simulink model "f_cd_reorder"  (R2018a)
settings: Solver=VariableStepAuto  StartTime=0.0  StopTime=200000  RelTol=1e-3
libraries: xbsIndex_r4 x1711, casper_library_misc x12, xps_library x2, simulink x1
(part 4 of 9)

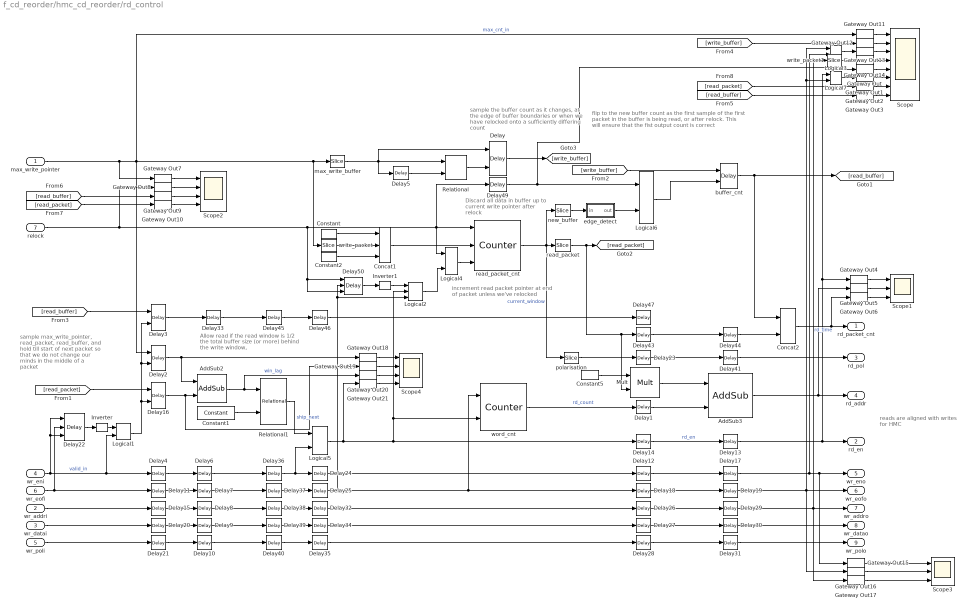
== system f_cd_reorder/hmc_cd_reorder/rd_control ==
  note: increment read packet pointer at
      | end of packet unless we've relocked
  note: flip to the new buffer count as the first sample of the
      | first packet in the buffer is being read, or after relock.
      | This will ensure that the fist output count is correct
  note: reads are aligned
      | with writes for HMC
  note: sample max_write_pointer,
      | read_packet, read_buffer,
      | and hold till start of
      | next packet so that
      | we do not change
      | our minds in the middle
      | of a packet
  note: sample the buffer count as it changes,
      | at the edge of buffer boundaries
      | or when we have relocked onto a
      | sufficiently differing count
  note: Allow read if the read window is 1/2
      | the total buffer size (or more)
      | behind the write window,
  note: Discard all data in buffer
      | up to current write pointer
      | after relock
  max_write_pointer : Inport
  wr_addri : Inport  Port=2
  wr_datai : Inport  Port=3
  wr_eni : Inport  Port=4
  wr_poli : Inport  Port=5
  wr_eofi : Inport  Port=6
  relock : Inport  Port=7
  AddSub2 : xbsIndex_r4/AddSub  mode=Subtraction  use_carryin=off  use_carryout=off  en=off  latency=1  precision=User Defined  arith_type=Unsigned  n_bits=n_bits_packets  bin_pt=0  quantization=Truncate  overflow=Wrap  use_behavioral_HDL=on  hw_selection=Fabric  pipelined=off  use_rpm=on  dbl_ovrd=off  block_type=addsub
      settings: xl_area=[0, 0, 0, 0, 0, 0, 0]  block_version=10.1.3
  AddSub3 : xbsIndex_r4/AddSub  mode=Addition  use_carryin=off  use_carryout=off  en=off  latency=1  precision=User Defined  arith_type=Unsigned  n_bits=n_bits_buffer_size-1  bin_pt=0  quantization=Truncate  overflow=Wrap  use_behavioral_HDL=on  hw_selection=Fabric  pipelined=off  use_rpm=on  dbl_ovrd=off  block_type=addsub
      settings: xl_area=[0, 0, 0, 0, 0, 0, 0]  block_version=10.1.3
  Concat1 : xbsIndex_r4/Concat  num_inputs=3  dbl_ovrd=off  block_type=concat
      settings: block_version=10.1.3
  Concat2 : xbsIndex_r4/Concat  num_inputs=2  dbl_ovrd=off  block_type=concat
      settings: block_version=10.1.3
  Constant : xbsIndex_r4/Constant  const=0  gui_display_data_type=Fixed-point  arith_type=Unsigned  n_bits=1  bin_pt=0  preci_type=Single  exp_width=8  frac_width=24  explicit_period=on  period=1  equ=P=C  opselect=C  inp2=PCIN>>17  opr=+  inp1=P  carry=CIN  dbl_ovrd=off  block_type=constant
  Constant1 : xbsIndex_r4/Constant  const=2^(n_bits_packets - 1)  gui_display_data_type=Fixed-point  arith_type=Unsigned  n_bits=n_bits_packets  bin_pt=0  preci_type=Single  exp_width=8  frac_width=24  explicit_period=on  period=1  equ=P=C  opselect=C  inp2=PCIN>>17  opr=+  inp1=P  carry=CIN  dbl_ovrd=off  block_type=constant
  Constant2 : xbsIndex_r4/Constant  const=0  gui_display_data_type=Fixed-point  arith_type=Unsigned  n_bits=1  bin_pt=0  preci_type=Single  exp_width=8  frac_width=24  explicit_period=on  period=1  equ=P=C  opselect=C  inp2=PCIN>>17  opr=+  inp1=P  carry=CIN  dbl_ovrd=off  block_type=constant
  Constant5 : xbsIndex_r4/Constant  const=packet_size  gui_display_data_type=Fixed-point  arith_type=Unsigned  n_bits=ceil(log2(packet_size))+1  bin_pt=0  preci_type=Single  exp_width=8  frac_width=24  explicit_period=on  period=1  equ=P=C  opselect=C  inp2=PCIN>>17  opr=+  inp1=P  carry=CIN  dbl_ovrd=off  block_type=constant
  Delay{,2..3,16} (4 alike) : xbsIndex_r4/Delay  rst=off  infoeditControl=Selection of Reset will increase slice count due to use of real FFs and instead of SRLs  en=on  latency=1  reg_retiming=on  dbl_ovrd=off  block_type=delay
      Delay16 settings: xl_area=[0, 0, 0, 0, 0, 0, 0]
      Delay2 settings: xl_area=[0, 0, 0, 0, 0, 0, 0]
      Delay3 settings: xl_area=[0, 0, 0, 0, 0, 0, 0]
  Delay{1,12,14,18,23,26..28,43,47} (10 alike) : xbsIndex_r4/Delay  rst=off  infoeditControl=Selection of Reset will increase slice count due to use of real FFs and instead of SRLs  en=off  latency=2  reg_retiming=on  dbl_ovrd=off  block_type=delay
      settings: xl_area=[0, 0, 0, 0, 0, 0, 0]
  Delay{4..11,13,15,17,19..21,24..25,29..41,44..46,49} (33 alike) : xbsIndex_r4/Delay  rst=off  infoeditControl=Selection of Reset will increase slice count due to use of real FFs and instead of SRLs  en=off  latency=1  reg_retiming=on  dbl_ovrd=off  block_type=delay
      Delay10 settings: xl_area=[0, 0, 0, 0, 0, 0, 0]
      Delay11 settings: xl_area=[0, 0, 0, 0, 0, 0, 0]
      Delay13 settings: infoedit=Hardware notes: A delay line is a chain, each link of which is an SRL16 or SRL32 followed by a flip-flop.  xl_area=[0, 0, 0, 0, 0, 0, 0]
      Delay15 settings: xl_area=[0, 0, 0, 0, 0, 0, 0]
      Delay17 settings: infoedit=Hardware notes: A delay line is a chain, each link of which is an SRL16 or SRL32 followed by a flip-flop.  xl_area=[0, 0, 0, 0, 0, 0, 0]
      Delay19 settings: infoedit=Hardware notes: A delay line is a chain, each link of which is an SRL16 or SRL32 followed by a flip-flop.  xl_area=[0, 0, 0, 0, 0, 0, 0]
      Delay20 settings: xl_area=[0, 0, 0, 0, 0, 0, 0]
      Delay21 settings: xl_area=[0, 0, 0, 0, 0, 0, 0]
      Delay24 settings: xl_area=[0, 0, 0, 0, 0, 0, 0]
      Delay25 settings: xl_area=[0, 0, 0, 0, 0, 0, 0]
      Delay29 settings: infoedit=Hardware notes: A delay line is a chain, each link of which is an SRL16 or SRL32 followed by a flip-flop.  xl_area=[0, 0, 0, 0, 0, 0, 0]
      Delay30 settings: infoedit=Hardware notes: A delay line is a chain, each link of which is an SRL16 or SRL32 followed by a flip-flop.  xl_area=[0, 0, 0, 0, 0, 0, 0]
      Delay31 settings: infoedit=Hardware notes: A delay line is a chain, each link of which is an SRL16 or SRL32 followed by a flip-flop.  xl_area=[0, 0, 0, 0, 0, 0, 0]
      Delay32 settings: xl_area=[0, 0, 0, 0, 0, 0, 0]
      Delay33 settings: xl_area=[0, 0, 0, 0, 0, 0, 0]
      Delay34 settings: xl_area=[0, 0, 0, 0, 0, 0, 0]
      Delay35 settings: xl_area=[0, 0, 0, 0, 0, 0, 0]
      Delay36 settings: xl_area=[0, 0, 0, 0, 0, 0, 0]
      Delay37 settings: xl_area=[0, 0, 0, 0, 0, 0, 0]
      Delay38 settings: xl_area=[0, 0, 0, 0, 0, 0, 0]
      Delay39 settings: xl_area=[0, 0, 0, 0, 0, 0, 0]
      Delay4 settings: xl_area=[0, 0, 0, 0, 0, 0, 0]
      Delay40 settings: xl_area=[0, 0, 0, 0, 0, 0, 0]
      Delay41 settings: infoedit=Hardware notes: A delay line is a chain, each link of which is an SRL16 or SRL32 followed by a flip-flop.  xl_area=[0, 0, 0, 0, 0, 0, 0]
      Delay44 settings: infoedit=Hardware notes: A delay line is a chain, each link of which is an SRL16 or SRL32 followed by a flip-flop.  xl_area=[0, 0, 0, 0, 0, 0, 0]
      Delay45 settings: xl_area=[0, 0, 0, 0, 0, 0, 0]
      Delay46 settings: xl_area=[0, 0, 0, 0, 0, 0, 0]
      Delay49 settings: xl_area=[0, 0, 0, 0, 0, 0, 0]
      Delay5 settings: xl_area=[0, 0, 0, 0, 0, 0, 0]
      Delay6 settings: xl_area=[0, 0, 0, 0, 0, 0, 0]
      Delay7 settings: xl_area=[0, 0, 0, 0, 0, 0, 0]
      Delay8 settings: xl_area=[0, 0, 0, 0, 0, 0, 0]
      Delay9 settings: xl_area=[0, 0, 0, 0, 0, 0, 0]
  Delay22 : xbsIndex_r4/Delay  rst=on  infoeditControl=Selection of Reset will increase slice count due to use of real FFs and instead of SRLs  en=on  latency=1  reg_retiming=on  dbl_ovrd=off  block_type=delay
      settings: xl_area=[0, 0, 0, 0, 0, 0, 0]
  Delay50 : xbsIndex_r4/Delay  rst=on  infoeditControl=Selection of Reset will increase slice count due to use of real FFs and instead of SRLs  en=on  latency=1  reg_retiming=on  dbl_ovrd=off  block_type=delay
      settings: xl_area=[0, 0, 0, 0, 0, 0, 0]
  Gateway Out{,1..21} (22 alike) : xbsIndex_r4/Gateway Out  inherit_from_input=off  hdl_port=off  rows=1  columns=1  UseAsDAC=off  DACChannel='1'  interface=None  automatic_assignment=on  address_offset=hex2dec('00')  intf_name=''  intf_description=''  timing_constraint=None  locs_specified=off  LOCs={}  io_standard={}  block_type=gatewayout
  Inverter : xbsIndex_r4/Inverter  en=off  latency=0  dbl_ovrd=off  block_type=inv
  Inverter1 : xbsIndex_r4/Inverter  en=off  latency=0  dbl_ovrd=off  block_type=inv
  Logical1 : xbsIndex_r4/Logical  logical_function=AND  inputs=2  en=off  latency=0  precision=Full  arith_type=Unsigned  n_bits=8  bin_pt=2  align_bp=on  dbl_ovrd=off  block_type=logical
      settings: xl_area=[0, 0, 0, 0, 0, 0, 0]
  Logical2 : xbsIndex_r4/Logical  logical_function=AND  inputs=3  en=off  latency=0  precision=Full  arith_type=Unsigned  n_bits=8  bin_pt=2  align_bp=on  dbl_ovrd=off  block_type=logical
      settings: xl_area=[0, 0, 0, 0, 0, 0, 0]
  Logical3 : xbsIndex_r4/Logical  logical_function=AND  inputs=2  en=off  latency=0  precision=Full  arith_type=Unsigned  n_bits=8  bin_pt=2  align_bp=on  dbl_ovrd=off  block_type=logical
      settings: xl_area=[0, 0, 0, 0, 0, 0, 0]
  Logical4 : xbsIndex_r4/Logical  logical_function=OR  inputs=2  en=off  latency=0  precision=Full  arith_type=Unsigned  n_bits=8  bin_pt=2  align_bp=on  dbl_ovrd=off  block_type=logical
      settings: xl_area=[0, 0, 0, 0, 0, 0, 0]
  Logical5 : xbsIndex_r4/Logical  logical_function=AND  inputs=2  en=off  latency=1  precision=Full  arith_type=Unsigned  n_bits=8  bin_pt=2  align_bp=on  dbl_ovrd=off  block_type=logical
      settings: xl_area=[0, 0, 0, 0, 0, 0, 0]
  Logical6 : xbsIndex_r4/Logical  logical_function=OR  inputs=2  en=off  latency=2  precision=Full  arith_type=Unsigned  n_bits=8  bin_pt=2  align_bp=on  dbl_ovrd=off  block_type=logical
      settings: xl_area=[0, 0, 0, 0, 0, 0, 0]
  Logical7 : xbsIndex_r4/Logical  logical_function=AND  inputs=2  en=off  latency=0  precision=Full  arith_type=Unsigned  n_bits=8  bin_pt=2  align_bp=on  dbl_ovrd=off  block_type=logical
      settings: xl_area=[0, 0, 0, 0, 0, 0, 0]
  Mult : xbsIndex_r4/Mult  precision=User Defined  arith_type=Unsigned  n_bits=n_bits_buffer_size-1  bin_pt=0  quantization=Truncate  overflow=Wrap  en=off  latency=2  use_behavioral_HDL=on  opt=Speed  use_embedded=on  optimum_pipeline=off  pipeline=on  dbl_ovrd=off  use_rpm=on  placement_style=Triangular  block_type=mult
  Relational : xbsIndex_r4/Relational  mode=a!=b  op_type=Bool  en=off  latency=0  dbl_ovrd=off  block_type=relational
  Relational1 : xbsIndex_r4/Relational  mode=a>=b  op_type=Bool  en=off  latency=1  dbl_ovrd=off  block_type=relational
      settings: xl_area=[0, 0, 0, 0, 0, 0, 0]  block_version=10.1.3
  Scope : Scope  NumInputPorts=8
  Scope1 : Scope  NumInputPorts=3
  Scope2 : Scope  NumInputPorts=4
  Scope3 : Scope  NumInputPorts=3
  Scope4 : Scope  NumInputPorts=4
  buffer_cnt : xbsIndex_r4/Delay  rst=off  infoeditControl=Selection of Reset will increase slice count due to use of real FFs and instead of SRLs  en=on  latency=1  reg_retiming=on  dbl_ovrd=off  block_type=delay
  edge_detect : Subsystem  AncestorBlock=casper_library_misc/edge_detect  mask(edge_detect){edge=Both, polarity=Active High, x_in=[0 0.08 0.08 0.16 0.16 0.24 0.24 0.32 0.32 0.4], y_in=[-1 -1  1  1  1  1  1  1  1  1], x_out=[0.6 0.68 0.68 0.76 0.76 0.84 0.84 0.92 0.92 1], y_out=[-1 -1  1  1 -1 -1 -1 -1 -1 -1]}
      mask prompts: edge "Edge Type"; polarity "Output Polarity"; x_in "Input X Positions"; y_in "Input Y Positions"; x_out "Output X Positions"; y_out "Output Y Positions"
      mask help: Output is active for one-cycle after each edge of the specified type (i.e. rising, falling or both).
      mask init: same as f_cd_reorder/data_width_convert/edge_detect
      settings: AttributesFormatString=|
      | both edges
      | active high
      mask Help: Output is active for one-cycle after each edge of the specified type (i.e. rising, falling, or both).  Latency is zero.
      mask TypeOptions edge: Rising | Falling | Both
      mask TypeOptions polarity: Active High | Active Low
      mask Display:
      | plot(x_in_num,0.5+y_in_num*0.2);
      | plot(x_out_num,0.5+y_out_num*0.2);
  max_write_buffer : xbsIndex_r4/Slice  nbits=1  boolean_output=off  mode=Two Bit Locations  bit1=0  base1=MSB of Input  bit0=n_bits_packets  base0=LSB of Input  dbl_ovrd=off  block_type=slice
      settings: block_version=10.1.3
  new_buffer : xbsIndex_r4/Slice  nbits=1  boolean_output=on  mode=Upper Bit Location + Width  bit1=0  base1=MSB of Input  bit0=0  base0=LSB of Input  dbl_ovrd=off  block_type=slice
  polarisation : xbsIndex_r4/Slice  nbits=1  boolean_output=off  mode=Lower Bit Location + Width  bit1=0  base1=MSB of Input  bit0=0  base0=LSB of Input  dbl_ovrd=off  block_type=slice
  read_packet : xbsIndex_r4/Slice  nbits=n_bits_packets  boolean_output=off  mode=Lower Bit Location + Width  bit1=0  base1=MSB of Input  bit0=1  base0=LSB of Input  dbl_ovrd=off  block_type=slice
  read_packet_cnt : xbsIndex_r4/Counter  cnt_type=Free Running  cnt_to=Inf  operation=Up  start_count=0  cnt_by_val=1  arith_type=Unsigned  n_bits=1+n_bits_packets+1  bin_pt=0  load_pin=on  rst=off  en=on  explicit_period=off  period=1  use_behavioral_HDL=off  implementation=Fabric  use_rpm=on  dbl_ovrd=off  block_type=counter
      settings: xl_area=[0, 0, 0, 0, 0, 0, 0]
  word_cnt : xbsIndex_r4/Counter  cnt_type=Count Limited  cnt_to=packet_size-1  operation=Up  start_count=0  cnt_by_val=1  arith_type=Unsigned  n_bits=ceil(log2(packet_size))  bin_pt=0  load_pin=off  rst=on  en=on  explicit_period=off  period=1  use_behavioral_HDL=on  implementation=Fabric  use_rpm=on  dbl_ovrd=off  block_type=counter
      settings: xl_area=[0, 0, 0, 0, 0, 0, 0]
  write_packet : xbsIndex_r4/Slice  nbits=n_bits_packets  boolean_output=off  mode=Lower Bit Location + Width  bit1=0  base1=MSB of Input  bit0=0  base0=LSB of Input  dbl_ovrd=off  block_type=slice
      settings: block_version=10.1.3
  write_packet1 : xbsIndex_r4/Slice  nbits=n_bits_packets  boolean_output=off  mode=Lower Bit Location + Width  bit1=0  base1=MSB of Input  bit0=ceil(log2(packet_size))  base0=LSB of Input  dbl_ovrd=off  block_type=slice
      settings: block_version=10.1.3
  rd_packet_cnt : Outport
  rd_en : Outport  Port=2
  rd_pol : Outport  Port=3
  rd_addr : Outport  Port=4
  wr_eno : Outport  Port=5
  wr_eofo : Outport  Port=6
  wr_addro : Outport  Port=7
  wr_datao : Outport  Port=8
  wr_polo : Outport  Port=9
  wires:
  read_packet/1 -> [read_packet], Delay43/1, Mult/2
  Constant1/1 -> Relational1/2
  AddSub2/1 -> Gateway Out20/1, Relational1/1  "win_lag"
  read_packet_cnt/1 -> new_buffer/1, polarisation/1, read_packet/1  "current_window"
  Concat2/1 -> rd_packet_cnt/1, Gateway Out6/1  "rd_time"
  max_write_pointer/1 -> max_write_buffer/1, write_packet/1, Gateway Out11/1, Delay2/1, Gateway Out7/1  "max_cnt_in"
  Relational1/1 -> Logical5/1  "ship_next"
  word_cnt/1 -> Delay1/1  "rd_count"
  Delay14/1 -> Delay13/1  "rd_en"
  Constant5/1 -> Mult/1
  Mult/1 -> AddSub3/1
  Delay1/1 -> AddSub3/2
  wr_eni/1 -> Logical1/2, Delay4/1, Delay22/3, Delay22/1  "valid_in"
  Relational/1 -> Delay/2
  Delay5/1 -> Relational/2
  Delay12/1 -> Delay17/1
  Delay13/1 -> rd_en/1, Logical7/1, Gateway Out4/1
  Delay17/1 -> wr_eno/1, Gateway Out15/1, Logical3/2
  Delay18/1 -> Delay19/1
  Delay26/1 -> Delay29/1
  Delay27/1 -> Delay30/1
  Delay28/1 -> Delay31/1
  Delay30/1 -> wr_datao/1
  Delay29/1 -> wr_addro/1, Gateway Out17/1, write_packet1/1
  Delay31/1 -> wr_polo/1
  Gateway Out6/1 -> Scope1/3
  Gateway Out5/1 -> Scope1/2
  Gateway Out4/1 -> Scope1/1
  wr_eofi/1 -> Delay22/2, Delay11/1
  wr_addri/1 -> Delay15/1
  wr_datai/1 -> Delay20/1
  wr_poli/1 -> Delay21/1
  Logical4/1 -> read_packet_cnt/3
  Logical2/1 -> Logical4/2
  max_write_buffer/1 -> Delay/1, Delay5/1, Relational/1
  Delay19/1 -> Logical7/2, Logical3/1, Gateway Out16/1, wr_eofo/1
  Delay6/1 -> Delay36/1
  Delay7/1 -> Delay37/1
  Delay8/1 -> Delay38/1
  Delay9/1 -> Delay39/1
  Delay10/1 -> Delay40/1
  Delay22/1 -> Inverter/1
  Inverter/1 -> Logical1/1
  [read_packet] -> Delay16/1
  Logical1/1 -> Delay3/2, Delay2/2, Delay16/2
  relock/1 -> Logical4/1, read_packet_cnt/1, Delay49/1, Delay50/1, Delay50/3, Gateway Out8/1
  Delay4/1 -> Delay6/1
  Delay11/1 -> Delay7/1
  Delay15/1 -> Delay8/1
  Delay20/1 -> Delay9/1
  Delay21/1 -> Delay10/1
  Logical5/1 -> word_cnt/2, Logical2/2, Delay14/1, Gateway Out21/1
  Delay24/1 -> Delay12/1
  Delay32/1 -> Delay26/1
  Delay34/1 -> Delay27/1
  Delay35/1 -> Delay28/1
  Delay36/1 -> Logical5/2, Delay24/1
  Delay37/1 -> Delay25/1
  Delay38/1 -> Delay32/1
  Delay39/1 -> Delay34/1
  Delay40/1 -> Delay35/1
  Delay2/1 -> AddSub2/1, Gateway Out18/1
  Delay16/1 -> Gateway Out19/1, AddSub2/2
  Delay43/1 -> Delay44/1
  Delay44/1 -> Concat2/2
  new_buffer/1 -> edge_detect/1(in)
  Logical6/1 -> buffer_cnt/2
  Delay/1 -> [write_buffer]
  [write_buffer] -> buffer_cnt/1
  [read_buffer] -> Delay3/1
  buffer_cnt/1 -> Concat2/1, [read_buffer]
  Delay46/1 -> Delay47/1
  Delay45/1 -> Delay46/1
  Delay33/1 -> Delay45/1
  Delay3/1 -> Delay33/1
  edge_detect/1(out) -> Logical6/2
  Delay49/1 -> Gateway Out/1, Logical6/1
  Gateway Out10/1 -> Scope2/4
  Gateway Out9/1 -> Scope2/3
  Gateway Out7/1 -> Scope2/1
  Gateway Out8/1 -> Scope2/2
  [read_buffer] -> Gateway Out9/1
  [read_packet] -> Gateway Out10/1
  Concat1/1 -> read_packet_cnt/2
  [read_buffer] -> Gateway Out3/1
  Gateway Out/1 -> Scope/5
  Gateway Out1/1 -> Scope/6
  Gateway Out2/1 -> Scope/7
  Gateway Out3/1 -> Scope/8
  Gateway Out11/1 -> Scope/1
  Gateway Out12/1 -> Scope/2
  Gateway Out13/1 -> Scope/3
  Gateway Out14/1 -> Scope/4
  [write_buffer] -> Gateway Out12/1
  [read_packet] -> Gateway Out2/1
  Gateway Out15/1 -> Scope3/1
  Gateway Out16/1 -> Scope3/2
  Gateway Out17/1 -> Scope3/3
  Logical3/1 -> Gateway Out13/1
  Logical7/1 -> Gateway Out1/1
  write_packet1/1 -> Gateway Out14/1
  Delay50/1 -> Inverter1/1
  Inverter1/1 -> Logical2/1
  Gateway Out18/1 -> Scope4/1
  Gateway Out19/1 -> Scope4/2
  Gateway Out20/1 -> Scope4/3
  Gateway Out21/1 -> Scope4/4
  Delay25/1 -> Logical2/3, Delay50/2, word_cnt/1, Delay18/1
  Constant/1 -> Concat1/1
  write_packet/1 -> Concat1/2
  AddSub3/1 -> rd_addr/1, Gateway Out5/1
  polarisation/1 -> Delay23/1
  Delay23/1 -> Delay41/1
  Delay41/1 -> rd_pol/1
  Constant2/1 -> Concat1/3

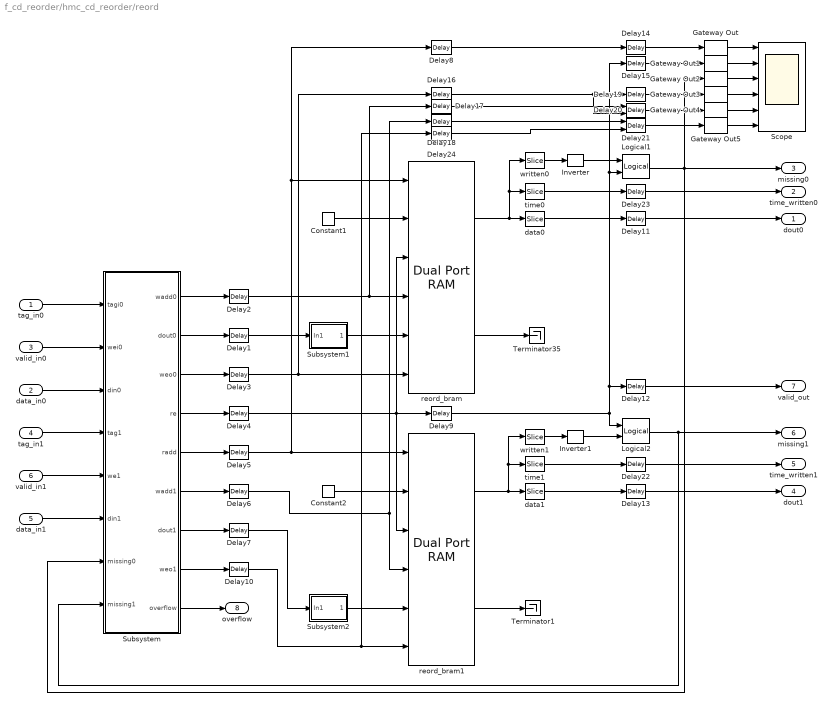
== system f_cd_reorder/hmc_cd_reorder/reord ==
  tag_in0 : Inport
  data_in0 : Inport  Port=2
  valid_in0 : Inport  Port=3
  tag_in1 : Inport  Port=4
  data_in1 : Inport  Port=5
  valid_in1 : Inport  Port=6
  Constant1 : xbsIndex_r4/Constant  const=0  gui_display_data_type=Fixed-point  arith_type=Unsigned  n_bits=80+1+n_bits_timestamp  bin_pt=0  preci_type=Single  exp_width=8  frac_width=24  explicit_period=on  period=1  equ=P=C  opselect=C  inp2=PCIN>>17  opr=+  inp1=P  carry=CIN  dbl_ovrd=off  block_type=constant
  Constant2 : xbsIndex_r4/Constant  const=0  gui_display_data_type=Fixed-point  arith_type=Unsigned  n_bits=80+1+n_bits_timestamp  bin_pt=0  preci_type=Single  exp_width=8  frac_width=24  explicit_period=on  period=1  equ=P=C  opselect=C  inp2=PCIN>>17  opr=+  inp1=P  carry=CIN  dbl_ovrd=off  block_type=constant
  Delay{1..7,10..15,19,22..23} (16 alike) : xbsIndex_r4/Delay  rst=off  infoeditControl=Selection of Reset will increase slice count due to use of real FFs and instead of SRLs  en=off  latency=1  reg_retiming=off  dbl_ovrd=off  block_type=delay
  Delay{8..9,16..18,24} (6 alike) : xbsIndex_r4/Delay  rst=off  infoeditControl=Selection of Reset will increase slice count due to use of real FFs and instead of SRLs  en=off  latency=bram_latency  reg_retiming=on  dbl_ovrd=off  block_type=delay
      settings: block_version=11.4
  Delay20 : xbsIndex_r4/Delay  rst=off  infoeditControl=Selection of Reset will increase slice count due to use of real FFs and instead of SRLs  en=on  latency=1  reg_retiming=off  dbl_ovrd=off  block_type=delay
  Delay21 : xbsIndex_r4/Delay  rst=off  infoeditControl=Selection of Reset will increase slice count due to use of real FFs and instead of SRLs  en=on  latency=1  reg_retiming=off  dbl_ovrd=off  block_type=delay
  Gateway Out{,1..5} (6 alike) : xbsIndex_r4/Gateway Out  inherit_from_input=off  hdl_port=off  rows=1  columns=1  UseAsDAC=off  DACChannel='1'  interface=None  automatic_assignment=on  address_offset=hex2dec('00')  intf_name=''  intf_description=''  timing_constraint=None  locs_specified=off  LOCs={}  io_standard={}  block_type=gatewayout
  Inverter : xbsIndex_r4/Inverter  en=off  latency=0  dbl_ovrd=off  block_type=inv
  Inverter1 : xbsIndex_r4/Inverter  en=off  latency=0  dbl_ovrd=off  block_type=inv
  Logical1 : xbsIndex_r4/Logical  logical_function=AND  inputs=2  en=off  latency=1  precision=Full  arith_type=Unsigned  n_bits=16  bin_pt=0  align_bp=on  dbl_ovrd=off  block_type=logical
  Logical2 : xbsIndex_r4/Logical  logical_function=AND  inputs=2  en=off  latency=1  precision=Full  arith_type=Unsigned  n_bits=16  bin_pt=0  align_bp=on  dbl_ovrd=off  block_type=logical
  Scope : Scope  NumInputPorts=6
  Subsystem : Subsystem
  Subsystem1 : Subsystem
  Subsystem2 : Subsystem
  Terminator1 : Terminator
  Terminator35 : Terminator
  data0 : xbsIndex_r4/Slice  nbits=80  boolean_output=off  mode=Lower Bit Location + Width  bit1=0  base1=MSB of Input  bit0=0  base0=LSB of Input  dbl_ovrd=off  block_type=slice
  data1 : xbsIndex_r4/Slice  nbits=80  boolean_output=off  mode=Lower Bit Location + Width  bit1=0  base1=MSB of Input  bit0=0  base0=LSB of Input  dbl_ovrd=off  block_type=slice
  reord_bram : xbsIndex_r4/Dual Port RAM  depth=2^n_bits_buffer  initVector=zeros(1,n_bits_buffer)  distributed_mem=Block RAM  init_a=0  init_b=0  rst_a=off  rst_b=off  en_a=off  en_b=off  latency=bram_latency  write_mode_A=Read Before Write  write_mode_B=Read Before Write  optimize=Speed  dbl_ovrd=off  block_type=dpram
  reord_bram1 : xbsIndex_r4/Dual Port RAM  depth=2^n_bits_buffer  initVector=zeros(1,n_bits_buffer)  distributed_mem=Block RAM  init_a=0  init_b=0  rst_a=off  rst_b=off  en_a=off  en_b=off  latency=bram_latency  write_mode_A=Read Before Write  write_mode_B=Read Before Write  optimize=Speed  dbl_ovrd=off  block_type=dpram
  time0 : xbsIndex_r4/Slice  nbits=n_bits_timestamp  boolean_output=off  mode=Lower Bit Location + Width  bit1=0  base1=MSB of Input  bit0=80  base0=LSB of Input  dbl_ovrd=off  block_type=slice
  time1 : xbsIndex_r4/Slice  nbits=n_bits_timestamp  boolean_output=off  mode=Lower Bit Location + Width  bit1=0  base1=MSB of Input  bit0=80  base0=LSB of Input  dbl_ovrd=off  block_type=slice
  written0 : xbsIndex_r4/Slice  nbits=1  boolean_output=on  mode=Upper Bit Location + Width  bit1=0  base1=MSB of Input  bit0=0  base0=LSB of Input  dbl_ovrd=off  block_type=slice
  written1 : xbsIndex_r4/Slice  nbits=1  boolean_output=on  mode=Upper Bit Location + Width  bit1=0  base1=MSB of Input  bit0=0  base0=LSB of Input  dbl_ovrd=off  block_type=slice
  dout0 : Outport
  time_written0 : Outport  Port=2
  missing0 : Outport  Port=3
  dout1 : Outport  Port=4
  time_written1 : Outport  Port=5
  missing1 : Outport  Port=6
  valid_out : Outport  Port=7
  overflow : Outport  Port=8
  wires:
  reord_bram1/2 -> Terminator1/1
  Constant1/1 -> reord_bram/2
  reord_bram/2 -> Terminator35/1
  data_in1/1 -> Subsystem/6(din1)
  tag_in0/1 -> Subsystem/1(tagi0)
  valid_in0/1 -> Subsystem/2(wei0)
  data_in0/1 -> Subsystem/3(din0)
  tag_in1/1 -> Subsystem/4(tag1)
  valid_in1/1 -> Subsystem/5(we1)
  Subsystem/1(wadd0) -> Delay2/1
  Subsystem/3(weo0) -> Delay3/1
  Subsystem/2(dout0) -> Delay1/1
  Subsystem/6(wadd1) -> Delay6/1
  Subsystem/8(weo1) -> Delay10/1
  Subsystem/7(dout1) -> Delay7/1
  Subsystem/4(re) -> Delay4/1
  Delay4/1 -> Delay9/1, reord_bram1/3, reord_bram/3
  Subsystem/5(radd) -> Delay5/1
  Delay2/1 -> Delay17/1, reord_bram/4
  Delay3/1 -> Delay16/1, reord_bram/6
  written0/1 -> Inverter/1
  written1/1 -> Inverter1/1
  Delay12/1 -> valid_out/1
  Subsystem2/1(Out1) -> reord_bram1/5
  Delay1/1 -> Subsystem1/1(In1)
  Subsystem1/1(Out1) -> reord_bram/5
  Delay7/1 -> Subsystem2/1(In1)
  reord_bram/1 -> written0/1, time0/1, data0/1
  reord_bram1/1 -> written1/1, time1/1, data1/1
  Delay9/1 -> Delay15/1, Logical1/2, Delay12/1, Logical2/1
  Delay10/1 -> Delay24/1, reord_bram1/6
  Delay6/1 -> Delay18/1, reord_bram1/4
  Delay5/1 -> reord_bram1/1, Delay8/1, reord_bram/1
  Constant2/1 -> reord_bram1/2
  Gateway Out/1 -> Scope/1
  Gateway Out2/1 -> Scope/3
  Gateway Out1/1 -> Scope/2
  Delay8/1 -> Delay14/1
  Delay14/1 -> Gateway Out/1
  Delay15/1 -> Gateway Out1/1
  Logical1/1 -> Subsystem/7(missing0), missing0/1, Gateway Out2/1
  Gateway Out3/1 -> Scope/4
  Gateway Out4/1 -> Scope/5
  Gateway Out5/1 -> Scope/6
  Delay16/1 -> Delay20/2, Delay19/1
  Delay17/1 -> Delay20/1
  Delay18/1 -> Delay21/1
  Delay21/1 -> Gateway Out5/1
  Delay19/1 -> Gateway Out3/1
  Delay20/1 -> Gateway Out4/1
  Inverter/1 -> Logical1/1
  Inverter1/1 -> Logical2/2
  Logical2/1 -> Subsystem/8(missing1), missing1/1
  Delay11/1 -> dout0/1
  data0/1 -> Delay11/1
  data1/1 -> Delay13/1
  Delay13/1 -> dout1/1
  time0/1 -> Delay23/1
  time1/1 -> Delay22/1
  Delay22/1 -> time_written1/1
  Delay23/1 -> time_written0/1
  Delay24/1 -> Delay21/2
  Subsystem/9(overflow) -> overflow/1

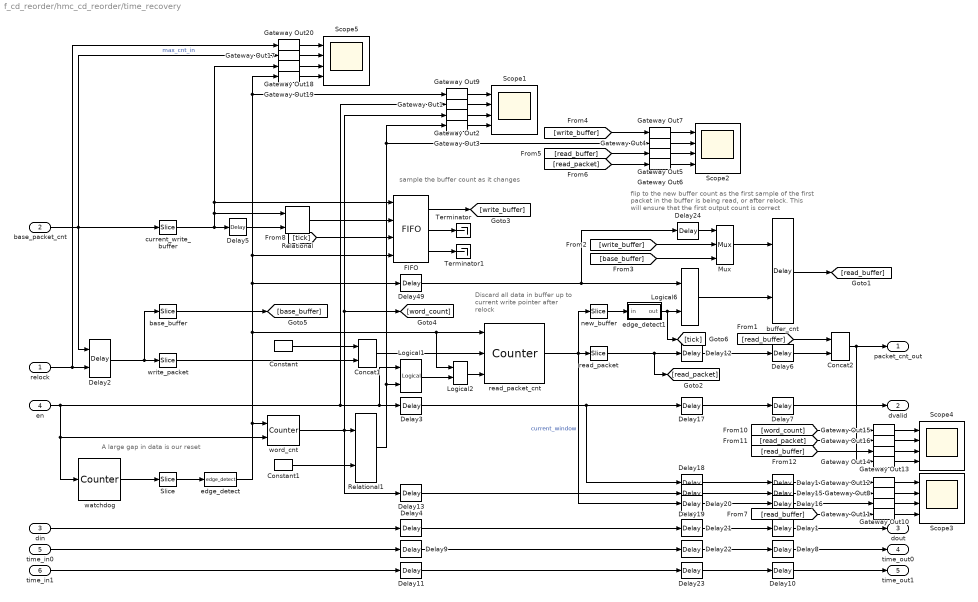
== system f_cd_reorder/hmc_cd_reorder/time_recovery ==
  note: A large gap in data is our reset
  note: Discard all data in buffer
      | up to current write pointer
      | after relock
  note: sample the buffer count as it changes
  note: flip to the new buffer count as the first sample of the
      | first packet in the buffer is being read, or after relock.
      | This will ensure that the first output count is correct
  relock : Inport
  base_packet_cnt : Inport  Port=2
  din : Inport  Port=3
  en : Inport  Port=4
  time_in0 : Inport  Port=5
  time_in1 : Inport  Port=6
  Concat1 : xbsIndex_r4/Concat  num_inputs=2  dbl_ovrd=off  block_type=concat
      settings: block_version=10.1.3
  Concat2 : xbsIndex_r4/Concat  num_inputs=2  dbl_ovrd=off  block_type=concat
      settings: block_version=10.1.3
  Constant : xbsIndex_r4/Constant  const=0  gui_display_data_type=Fixed-point  arith_type=Unsigned  n_bits=1  bin_pt=0  preci_type=Single  exp_width=8  frac_width=24  explicit_period=on  period=1  equ=P=C  opselect=C  inp2=PCIN>>17  opr=+  inp1=P  carry=CIN  dbl_ovrd=off  block_type=constant
  Constant1 : xbsIndex_r4/Constant  const=packet_size*2-1  gui_display_data_type=Fixed-point  arith_type=Unsigned  n_bits=ceil(log2(packet_size))+1  bin_pt=0  preci_type=Single  exp_width=8  frac_width=24  explicit_period=on  period=1  equ=P=C  opselect=C  inp2=PCIN>>17  opr=+  inp1=P  carry=CIN  dbl_ovrd=off  block_type=constant
  Delay{1,3..24,49} (24 alike) : xbsIndex_r4/Delay  rst=off  infoeditControl=Selection of Reset will increase slice count due to use of real FFs and instead of SRLs  en=off  latency=1  reg_retiming=on  dbl_ovrd=off  block_type=delay
      settings: xl_area=[0, 0, 0, 0, 0, 0, 0]
  Delay2 : xbsIndex_r4/Delay  rst=off  infoeditControl=Selection of Reset will increase slice count due to use of real FFs and instead of SRLs  en=on  latency=1  reg_retiming=on  dbl_ovrd=off  block_type=delay
      settings: xl_area=[0, 0, 0, 0, 0, 0, 0]
  FIFO : xbsIndex_r4/FIFO  mem_type=Distributed RAM  performance_options=Standard_FIFO  embedded_registers=off  depth=16  percent_nbits=1  rst=on  rst_latency=1  en=off  use_dcount=off  use_percent_full_port=off  use_almost_empty=off  almost_empty_thresh=2  use_almost_full=off  almost_full_thresh=14  explicit_period=off  dbl_ovrd=off  block_type=fifo
  Gateway Out{1..20} (20 alike) : xbsIndex_r4/Gateway Out  inherit_from_input=off  hdl_port=off  rows=1  columns=1  UseAsDAC=off  DACChannel='1'  interface=None  automatic_assignment=on  address_offset=hex2dec('00')  intf_name=''  intf_description=''  timing_constraint=None  locs_specified=off  LOCs={}  io_standard={}  block_type=gatewayout
  Logical1 : xbsIndex_r4/Logical  logical_function=AND  inputs=2  en=off  latency=1  precision=Full  arith_type=Unsigned  n_bits=8  bin_pt=2  align_bp=on  dbl_ovrd=off  block_type=logical
      settings: xl_area=[0, 0, 0, 0, 0, 0, 0]
  Logical2 : xbsIndex_r4/Logical  logical_function=OR  inputs=2  en=off  latency=0  precision=Full  arith_type=Unsigned  n_bits=8  bin_pt=2  align_bp=on  dbl_ovrd=off  block_type=logical
      settings: xl_area=[0, 0, 0, 0, 0, 0, 0]
  Logical6 : xbsIndex_r4/Logical  logical_function=OR  inputs=2  en=off  latency=1  precision=Full  arith_type=Unsigned  n_bits=8  bin_pt=2  align_bp=on  dbl_ovrd=off  block_type=logical
      settings: xl_area=[0, 0, 0, 0, 0, 0, 0]
  Mux : xbsIndex_r4/Mux  inputs=2  en=off  latency=0  precision=Full  arith_type=Unsigned  n_bits=16  bin_pt=14  quantization=Truncate  overflow=Wrap  dbl_ovrd=off  block_type=mux
  Relational : xbsIndex_r4/Relational  mode=a!=b  op_type=Bool  en=off  latency=0  dbl_ovrd=off  block_type=relational
  Relational1 : xbsIndex_r4/Relational  mode=a=b  op_type=Bool  en=off  latency=0  dbl_ovrd=off  block_type=relational
  Scope{1..5} (5 alike) : Scope  NumInputPorts=4
  Slice : xbsIndex_r4/Slice  nbits=1  boolean_output=on  mode=Upper Bit Location + Width  bit1=0  base1=MSB of Input  bit0=0  base0=LSB of Input  dbl_ovrd=off  block_type=slice
  Terminator : Terminator
  Terminator1 : Terminator
  base_buffer : xbsIndex_r4/Slice  nbits=1  boolean_output=off  mode=Two Bit Locations  bit1=0  base1=MSB of Input  bit0=n_bits_packets  base0=LSB of Input  dbl_ovrd=off  block_type=slice
      settings: block_version=10.1.3
  buffer_cnt : xbsIndex_r4/Delay  rst=off  infoeditControl=Selection of Reset will increase slice count due to use of real FFs and instead of SRLs  en=on  latency=1  reg_retiming=on  dbl_ovrd=off  block_type=delay
  current_write_buffer : xbsIndex_r4/Slice  nbits=1  boolean_output=off  mode=Two Bit Locations  bit1=0  base1=MSB of Input  bit0=n_bits_packets  base0=LSB of Input  dbl_ovrd=off  block_type=slice
      settings: block_version=10.1.3
  edge_detect : casper_library_misc/edge_detect  edge=Rising  polarity=Active High  x_in=[0 0.08 0.08 0.16 0.16 0.24 0.24 0.32 0.32 0.4]  y_in="[-1 -1  1  1  1  1  1  1  1  1]"  x_out=[0.6 0.68 0.68 0.76 0.76 0.84 0.84 0.92 0.92 1]  y_out="[-1 -1  1  1 -1 -1 -1 -1 -1 -1]"
  edge_detect1 : Subsystem  AncestorBlock=casper_library_misc/edge_detect  mask(edge_detect){edge=Both, polarity=Active High, x_in=[0 0.08 0.08 0.16 0.16 0.24 0.24 0.32 0.32 0.4], y_in=[-1 -1  1  1  1  1  1  1  1  1], x_out=[0.6 0.68 0.68 0.76 0.76 0.84 0.84 0.92 0.92 1], y_out=[-1 -1  1  1 -1 -1 -1 -1 -1 -1]}
      mask prompts: edge "Edge Type"; polarity "Output Polarity"; x_in "Input X Positions"; y_in "Input Y Positions"; x_out "Output X Positions"; y_out "Output Y Positions"
      mask help: Output is active for one-cycle after each edge of the specified type (i.e. rising, falling or both).
      mask init: same as f_cd_reorder/data_width_convert/edge_detect
      settings: AttributesFormatString=|
      | both edges
      | active high
      mask Help: Output is active for one-cycle after each edge of the specified type (i.e. rising, falling, or both).  Latency is zero.
      mask TypeOptions edge: Rising | Falling | Both
      mask TypeOptions polarity: Active High | Active Low
      mask Display:
      | plot(x_in_num,0.5+y_in_num*0.2);
      | plot(x_out_num,0.5+y_out_num*0.2);
  new_buffer : xbsIndex_r4/Slice  nbits=1  boolean_output=on  mode=Upper Bit Location + Width  bit1=0  base1=MSB of Input  bit0=0  base0=LSB of Input  dbl_ovrd=off  block_type=slice
  read_packet : xbsIndex_r4/Slice  nbits=n_bits_packets  boolean_output=off  mode=Lower Bit Location + Width  bit1=0  base1=MSB of Input  bit0=0  base0=LSB of Input  dbl_ovrd=off  block_type=slice
  read_packet_cnt : xbsIndex_r4/Counter  cnt_type=Free Running  cnt_to=Inf  operation=Up  start_count=0  cnt_by_val=1  arith_type=Unsigned  n_bits=n_bits_packets+1  bin_pt=0  load_pin=on  rst=off  en=on  explicit_period=off  period=1  use_behavioral_HDL=on  implementation=Fabric  use_rpm=on  dbl_ovrd=off  block_type=counter
      settings: xl_area=[0, 0, 0, 0, 0, 0, 0]
  watchdog : xbsIndex_r4/Counter  cnt_type=Free Running  cnt_to=Inf  operation=Up  start_count=0  cnt_by_val=1  arith_type=Unsigned  n_bits=n_bits_buffer_size-2  bin_pt=0  load_pin=off  rst=on  en=off  explicit_period=on  period=1  use_behavioral_HDL=off  implementation=Fabric  dbl_ovrd=off  block_type=counter
  word_cnt : xbsIndex_r4/Counter  cnt_type=Count Limited  cnt_to=packet_size*2-1  operation=Up  start_count=0  cnt_by_val=1  arith_type=Unsigned  n_bits=ceil(log2(packet_size))+1  bin_pt=0  load_pin=off  rst=on  en=on  explicit_period=off  period=1  use_behavioral_HDL=on  implementation=Fabric  use_rpm=on  dbl_ovrd=off  block_type=counter
      settings: xl_area=[0, 0, 0, 0, 0, 0, 0]
  write_packet : xbsIndex_r4/Slice  nbits=n_bits_packets  boolean_output=off  mode=Lower Bit Location + Width  bit1=0  base1=MSB of Input  bit0=0  base0=LSB of Input  dbl_ovrd=off  block_type=slice
      settings: block_version=10.1.3
  packet_cnt_out : Outport
  dvalid : Outport  Port=2
  dout : Outport  Port=3
  time_out0 : Outport  Port=4
  time_out1 : Outport  Port=5
  wires:
  Delay49/1 -> Delay24/1, Logical6/1
  edge_detect1/1(out) -> [tick], Logical6/2
  edge_detect/1 -> word_cnt/1, Logical2/1, read_packet_cnt/1, Gateway Out19/1, Gateway Out9/1, FIFO/4, Delay49/1
  FIFO/1 -> [write_buffer]
  relock/1 -> Gateway Out20/1, Delay2/2
  write_packet/1 -> Concat1/2
  Logical6/1 -> buffer_cnt/2
  read_packet/1 -> [read_packet], Delay12/1
  Delay5/1 -> Relational/2
  Relational/1 -> FIFO/2
  read_packet_cnt/1 -> Delay20/1, read_packet/1, new_buffer/1  "current_window"
  current_write_buffer/1 -> Gateway Out18/1, FIFO/1, Relational/1, Delay5/1
  Concat1/1 -> read_packet_cnt/2
  Constant/1 -> Concat1/1
  new_buffer/1 -> edge_detect1/1(in)
  Slice/1 -> edge_detect/1
  watchdog/1 -> Slice/1
  base_packet_cnt/1 -> Delay2/1, Gateway Out17/1, current_write_buffer/1  "max_cnt_in"
  Delay2/1 -> base_buffer/1, write_packet/1
  word_cnt/1 -> Delay13/1, Gateway Out2/1, [word_count], Relational1/1
  Constant1/1 -> Relational1/2
  en/1 -> Delay3/1, Logical1/1, Gateway Out1/1, watchdog/1, word_cnt/2
  Relational1/1 -> Gateway Out4/1, Gateway Out3/1, Logical1/2
  din/1 -> Delay4/1
  [read_buffer] -> Concat2/1
  Delay6/1 -> Concat2/2
  Concat2/1 -> packet_cnt_out/1, Gateway Out14/1
  Delay3/1 -> Delay18/1, Delay17/1
  Delay4/1 -> Delay21/1
  Gateway Out9/1 -> Scope1/1
  Gateway Out1/1 -> Scope1/2
  Gateway Out2/1 -> Scope1/3
  Gateway Out3/1 -> Scope1/4
  Gateway Out6/1 -> Scope2/4
  Gateway Out5/1 -> Scope2/3
  Gateway Out4/1 -> Scope2/2
  Gateway Out7/1 -> Scope2/1
  [write_buffer] -> Gateway Out7/1
  [read_buffer] -> Gateway Out5/1
  [read_packet] -> Gateway Out6/1
  Gateway Out12/1 -> Scope3/1
  Gateway Out8/1 -> Scope3/2
  Gateway Out10/1 -> Scope3/3
  Gateway Out11/1 -> Scope3/4
  Gateway Out14/1 -> Scope4/4
  Gateway Out13/1 -> Scope4/3
  Gateway Out16/1 -> Scope4/2
  Gateway Out15/1 -> Scope4/1
  [word_count] -> Gateway Out15/1
  [read_packet] -> Gateway Out16/1
  [read_buffer] -> Gateway Out13/1
  Delay7/1 -> dvalid/1
  Delay1/1 -> dout/1
  Delay11/1 -> Delay23/1
  Delay9/1 -> Delay22/1
  Delay8/1 -> time_out0/1
  Delay10/1 -> time_out1/1
  time_in0/1 -> Delay9/1
  time_in1/1 -> Delay11/1
  Gateway Out19/1 -> Scope5/4
  Gateway Out18/1 -> Scope5/3
  Gateway Out17/1 -> Scope5/2
  Gateway Out20/1 -> Scope5/1
  Mux/1 -> buffer_cnt/1
  [write_buffer] -> Mux/2
  base_buffer/1 -> [base_buffer]
  [base_buffer] -> Mux/3
  Logical2/1 -> read_packet_cnt/3
  Logical1/1 -> Logical2/2
  Delay13/1 -> Delay19/1
  [read_buffer] -> Gateway Out11/1
  Delay14/1 -> Gateway Out12/1
  Delay15/1 -> Gateway Out8/1
  Delay16/1 -> Gateway Out10/1
  FIFO/3 -> Terminator1/1
  FIFO/2 -> Terminator/1
  [tick] -> FIFO/3
  buffer_cnt/1 -> [read_buffer]
  Delay12/1 -> Delay6/1
  Delay17/1 -> Delay7/1
  Delay18/1 -> Delay14/1
  Delay19/1 -> Delay15/1
  Delay20/1 -> Delay16/1
  Delay21/1 -> Delay1/1
  Delay22/1 -> Delay8/1
  Delay23/1 -> Delay10/1
  Delay24/1 -> Mux/1

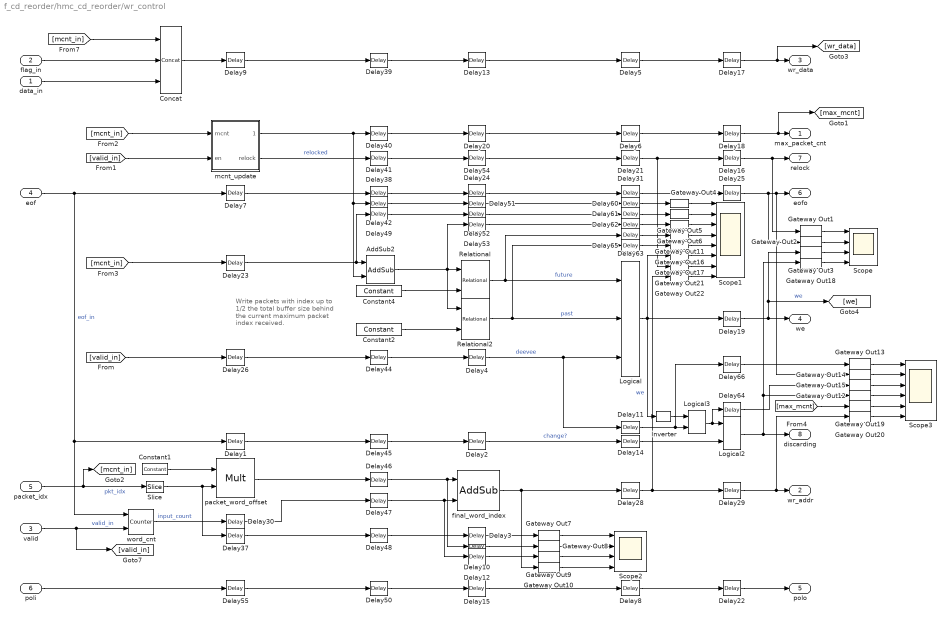
== system f_cd_reorder/hmc_cd_reorder/wr_control ==
  note: Write packets with index
      | up to 1/2 the total buffer size
      |  behind the current maximum
      | packet index received.
  data_in : Inport
  flag_in : Inport  Port=2
  valid : Inport  Port=3
  eof : Inport  Port=4
  packet_idx : Inport  Port=5
  poli : Inport  Port=6
  AddSub2 : xbsIndex_r4/AddSub  mode=Subtraction  use_carryin=off  use_carryout=off  en=off  latency=1  precision=Full  arith_type="Signed  (2's comp)"  n_bits=1  bin_pt=0  quantization=Truncate  overflow=Wrap  use_behavioral_HDL=off  hw_selection=Fabric  pipelined=on  use_rpm=on  dbl_ovrd=off  block_type=addsub
      settings: xl_area=[0, 0, 0, 0, 0, 0, 0]  block_version=10.1.3
  Concat : xbsIndex_r4/Concat  num_inputs=3  dbl_ovrd=off  block_type=concat
      settings: block_version=10.1.3
  Constant1 : xbsIndex_r4/Constant  const=packet_size  gui_display_data_type=Fixed-point  arith_type=Unsigned  n_bits=ceil(log2(packet_size))+1  bin_pt=0  preci_type=Single  exp_width=8  frac_width=24  explicit_period=on  period=1  equ=P=C  opselect=C  inp2=PCIN>>17  opr=+  inp1=P  carry=CIN  dbl_ovrd=off  block_type=constant
  Constant2 : xbsIndex_r4/Constant  const=0  gui_display_data_type=Fixed-point  arith_type=Signed (2's comp)  n_bits=n_bits_packets+1  bin_pt=0  preci_type=Single  exp_width=8  frac_width=24  explicit_period=on  period=1  equ=P=C  opselect=C  inp2=PCIN>>17  opr=+  inp1=P  carry=CIN  dbl_ovrd=off  block_type=constant
  Constant4 : xbsIndex_r4/Constant  const=-2^((n_bits_packets)-1)  gui_display_data_type=Fixed-point  arith_type=Signed (2's comp)  n_bits=n_bits_packets+1  bin_pt=0  preci_type=Single  exp_width=8  frac_width=24  explicit_period=on  period=1  equ=P=C  opselect=C  inp2=PCIN>>17  opr=+  inp1=P  carry=CIN  dbl_ovrd=off  block_type=constant
  Delay{1,7,9,23,26,30,37,55} (8 alike) : xbsIndex_r4/Delay  rst=off  infoeditControl=Selection of Reset will increase slice count due to use of real FFs and instead of SRLs  en=off  latency=3  reg_retiming=on  dbl_ovrd=off  block_type=delay
      settings: xl_area=[0, 0, 0, 0, 0, 0, 0]
  Delay{2..4,10,12..13,15,20,24,51..54} (13 alike) : xbsIndex_r4/Delay  rst=off  infoeditControl=Selection of Reset will increase slice count due to use of real FFs and instead of SRLs  en=off  latency=2  reg_retiming=on  dbl_ovrd=off  block_type=delay
      Delay10 settings: infoedit=Hardware notes: A delay line is a chain, each link of which is an SRL16 or SRL32 followed by a flip-flop.  xl_area=[0, 0, 0, 0, 0, 0, 0]
      Delay12 settings: infoedit=Hardware notes: A delay line is a chain, each link of which is an SRL16 or SRL32 followed by a flip-flop.  xl_area=[0, 0, 0, 0, 0, 0, 0]
      Delay13 settings: xl_area=[0, 0, 0, 0, 0, 0, 0]
      Delay15 settings: infoedit=Hardware notes: A delay line is a chain, each link of which is an SRL16 or SRL32 followed by a flip-flop.  xl_area=[0, 0, 0, 0, 0, 0, 0]
      Delay2 settings: xl_area=[0, 0, 0, 0, 0, 0, 0]
      Delay20 settings: xl_area=[0, 0, 0, 0, 0, 0, 0]
      Delay24 settings: infoedit=Hardware notes: A delay line is a chain, each link of which is an SRL16 or SRL32 followed by a flip-flop.  xl_area=[0, 0, 0, 0, 0, 0, 0]
      Delay3 settings: infoedit=Hardware notes: A delay line is a chain, each link of which is an SRL16 or SRL32 followed by a flip-flop.  xl_area=[0, 0, 0, 0, 0, 0, 0]
      Delay4 settings: infoedit=Hardware notes: A delay line is a chain, each link of which is an SRL16 or SRL32 followed by a flip-flop.  xl_area=[0, 0, 0, 0, 0, 0, 0]
      Delay51 settings: infoedit=Hardware notes: A delay line is a chain, each link of which is an SRL16 or SRL32 followed by a flip-flop.  xl_area=[0, 0, 0, 0, 0, 0, 0]
      Delay52 settings: infoedit=Hardware notes: A delay line is a chain, each link of which is an SRL16 or SRL32 followed by a flip-flop.  xl_area=[0, 0, 0, 0, 0, 0, 0]
      Delay53 settings: infoedit=Hardware notes: A delay line is a chain, each link of which is an SRL16 or SRL32 followed by a flip-flop.  xl_area=[0, 0, 0, 0, 0, 0, 0]
      Delay54 settings: xl_area=[0, 0, 0, 0, 0, 0, 0]
  Delay{5..6,8,11,14,16..19,21..22,25,28..29,31,38..42,44..50,60..66} (34 alike) : xbsIndex_r4/Delay  rst=off  infoeditControl=Selection of Reset will increase slice count due to use of real FFs and instead of SRLs  en=off  latency=1  reg_retiming=on  dbl_ovrd=off  block_type=delay
      settings: xl_area=[0, 0, 0, 0, 0, 0, 0]
  Gateway Out{1..22} (22 alike) : xbsIndex_r4/Gateway Out  inherit_from_input=off  hdl_port=off  rows=1  columns=1  UseAsDAC=off  DACChannel='1'  interface=None  automatic_assignment=on  address_offset=hex2dec('00')  intf_name=''  intf_description=''  timing_constraint=None  locs_specified=off  LOCs={}  io_standard={}  block_type=gatewayout
  Inverter : xbsIndex_r4/Inverter  en=off  latency=0  dbl_ovrd=off  block_type=inv
  Logical : xbsIndex_r4/Logical  logical_function=AND  inputs=3  en=off  latency=1  precision=Full  arith_type=Unsigned  n_bits=8  bin_pt=2  align_bp=on  dbl_ovrd=off  block_type=logical
      settings: xl_area=[0, 0, 0, 0, 0, 0, 0]
  Logical2 : xbsIndex_r4/Logical  logical_function=AND  inputs=2  en=off  latency=1  precision=Full  arith_type=Unsigned  n_bits=8  bin_pt=2  align_bp=on  dbl_ovrd=off  block_type=logical
      settings: xl_area=[0, 0, 0, 0, 0, 0, 0]
  Logical3 : xbsIndex_r4/Logical  logical_function=AND  inputs=2  en=off  latency=0  precision=Full  arith_type=Unsigned  n_bits=8  bin_pt=2  align_bp=on  dbl_ovrd=off  block_type=logical
      settings: xl_area=[0, 0, 0, 0, 0, 0, 0]
  Relational : xbsIndex_r4/Relational  mode=a>b  op_type=Bool  en=off  latency=2  dbl_ovrd=off  block_type=relational
      settings: xl_area=[0, 0, 0, 0, 0, 0, 0]  block_version=10.1.3
  Relational2 : xbsIndex_r4/Relational  mode=a<=b  op_type=Bool  en=off  latency=2  dbl_ovrd=off  block_type=relational
      settings: xl_area=[0, 0, 0, 0, 0, 0, 0]  block_version=10.1.3
  Scope : Scope  NumInputPorts=4
  Scope1 : Scope  NumInputPorts=8
  Scope2 : Scope  NumInputPorts=4
  Scope3 : Scope  NumInputPorts=6
  Slice : xbsIndex_r4/Slice  nbits=n_bits_packets  boolean_output=off  mode=Lower Bit Location + Width  bit1=0  base1=MSB of Input  bit0=0  base0=LSB of Input  dbl_ovrd=off  block_type=slice
  final_word_index : xbsIndex_r4/AddSub  mode=Addition  use_carryin=off  use_carryout=off  en=off  latency=2  precision=User Defined  arith_type=Unsigned  n_bits=n_bits_buffer_size  bin_pt=0  quantization=Truncate  overflow=Wrap  use_behavioral_HDL=off  hw_selection=Fabric  pipelined=off  dbl_ovrd=off  block_type=addsub
  mcnt_update : Subsystem
  packet_word_offset : xbsIndex_r4/Mult  precision=User Defined  arith_type=Unsigned  n_bits=n_bits_buffer_size  bin_pt=0  quantization=Truncate  overflow=Wrap  en=off  latency=3  use_behavioral_HDL=off  opt=Speed  use_embedded=on  optimum_pipeline=off  pipeline=on  dbl_ovrd=off  use_rpm=on  placement_style=Triangular  block_type=mult
  word_cnt : xbsIndex_r4/Counter  cnt_type=Free Running  cnt_to=Inf  operation=Up  start_count=0  cnt_by_val=1  arith_type=Unsigned  n_bits=ceil(log2(packet_size))  bin_pt=0  load_pin=off  rst=on  en=on  explicit_period=off  period=1  use_behavioral_HDL=off  implementation=Fabric  use_rpm=on  dbl_ovrd=off  block_type=counter
      settings: xl_area=[0, 0, 0, 0, 0, 0, 0]
  max_packet_cnt : Outport
  wr_addr : Outport  Port=2
  wr_data : Outport  Port=3
  we : Outport  Port=4
  polo : Outport  Port=5
  eofo : Outport  Port=6
  relock : Outport  Port=7
  discarding : Outport  Port=8
  wires:
  Delay20/1 -> Delay6/1
  Delay9/1 -> Delay39/1
  eof/1 -> Delay7/1, word_cnt/1, Delay1/1  "eof_in"
  Delay4/1 -> Delay11/1, Logical/3  "deevee"
  Logical/1 -> Gateway Out17/1, Delay19/1, Inverter/1  "we"
  valid/1 -> [valid_in], word_cnt/2  "valid_in"
  packet_idx/1 -> [mcnt_in], Slice/1  "pkt_idx"
  Delay13/1 -> Delay5/1
  Delay15/1 -> Delay8/1
  word_cnt/1 -> Delay30/1  "input_count"
  AddSub2/1 -> Delay53/1, Relational/1, Relational2/1
  mcnt_update/2(relock) -> Delay41/1  "relocked"
  Logical2/1 -> discarding/1, Gateway Out12/1, Gateway Out18/1
  Delay2/1 -> Delay14/1  "change?"
  Relational/1 -> Delay63/1, Logical/1  "future"
  Relational2/1 -> Delay65/1, Logical/2  "past"
  Delay5/1 -> Delay17/1
  Delay6/1 -> Delay18/1
  Delay8/1 -> Delay22/1
  Delay14/1 -> Logical2/2
  Delay17/1 -> [wr_data], wr_data/1
  Delay18/1 -> [max_mcnt], max_packet_cnt/1
  Delay19/1 -> we/1, [we], Gateway Out3/1  "we"
  Delay22/1 -> polo/1
  Delay55/1 -> Delay50/1
  Constant1/1 -> packet_word_offset/1
  packet_word_offset/1 -> Delay46/1
  final_word_index/1 -> Delay28/1, Gateway Out10/1
  Delay29/1 -> Gateway Out20/1, wr_addr/1
  Delay30/1 -> Delay47/1
  Delay26/1 -> Delay44/1
  [valid_in] -> Delay26/1
  [valid_in] -> mcnt_update/2(en)
  Delay16/1 -> Gateway Out1/1, relock/1
  Delay28/1 -> Delay29/1, Gateway Out22/1
  Delay7/1 -> Delay38/1
  Delay31/1 -> Delay25/1
  Delay24/1 -> Delay31/1
  Delay25/1 -> Gateway Out2/1, Gateway Out14/1, eofo/1
  Delay21/1 -> Gateway Out21/1, Delay16/1
  poli/1 -> Delay55/1
  Gateway Out5/1 -> Scope1/2
  Gateway Out4/1 -> Scope1/1
  Gateway Out6/1 -> Scope1/3
  Gateway Out10/1 -> Scope2/4
  Gateway Out8/1 -> Scope2/2
  Gateway Out7/1 -> Scope2/1
  Gateway Out9/1 -> Scope2/3
  Delay37/1 -> Delay48/1
  Delay10/1 -> Gateway Out8/1
  Delay3/1 -> Gateway Out7/1
  Delay12/1 -> Gateway Out9/1
  [mcnt_in] -> Delay23/1
  Delay38/1 -> Delay24/1
  Delay41/1 -> Delay54/1
  Delay40/1 -> Delay20/1
  Delay39/1 -> Delay13/1
  mcnt_update/1(maxcnt) -> Delay40/1, Delay42/1, AddSub2/2
  Delay23/1 -> AddSub2/1, Delay49/1
  Constant4/1 -> Relational/2
  Gateway Out11/1 -> Scope1/4
  Delay45/1 -> Delay2/1
  Delay44/1 -> Delay4/1
  Delay46/1 -> Delay10/1, final_word_index/1
  Delay47/1 -> Delay12/1, final_word_index/2
  Delay48/1 -> Delay3/1
  Delay42/1 -> Delay51/1
  Delay49/1 -> Delay52/1
  Delay51/1 -> Delay60/1
  Delay52/1 -> Delay61/1
  Delay53/1 -> Delay62/1
  [mcnt_in] -> mcnt_update/1(mcnt)
  Constant2/1 -> Relational2/2
  Delay50/1 -> Delay15/1
  Delay54/1 -> Delay21/1
  Gateway Out15/1 -> Scope3/3
  Gateway Out13/1 -> Scope3/1
  Gateway Out14/1 -> Scope3/2
  Gateway Out12/1 -> Scope3/4
  Delay65/1 -> Gateway Out16/1
  Delay60/1 -> Gateway Out4/1
  Delay61/1 -> Gateway Out5/1
  Delay62/1 -> Gateway Out6/1
  Delay63/1 -> Gateway Out11/1
  Gateway Out16/1 -> Scope1/5
  Gateway Out17/1 -> Scope1/6
  Slice/1 -> Delay37/1, packet_word_offset/2
  Gateway Out1/1 -> Scope/1
  Gateway Out18/1 -> Scope/4
  Gateway Out3/1 -> Scope/3
  Gateway Out2/1 -> Scope/2
  Inverter/1 -> Logical3/1
  Delay11/1 -> Delay66/1, Logical3/2
  Logical3/1 -> Delay64/1, Logical2/1
  Gateway Out19/1 -> Scope3/5
  Gateway Out20/1 -> Scope3/6
  Delay64/1 -> Gateway Out15/1
  Delay66/1 -> Gateway Out13/1
  Delay1/1 -> Delay45/1
  [max_mcnt] -> Gateway Out19/1
  Concat/1 -> Delay9/1
  data_in/1 -> Concat/3
  [mcnt_in] -> Concat/1
  flag_in/1 -> Concat/2
  Gateway Out21/1 -> Scope1/7
  Gateway Out22/1 -> Scope1/8

== system f_cd_reorder/munge2/join ==
  in1 : Inport
  in2 : Inport  Port=2
  in3 : Inport  Port=3
  in4 : Inport  Port=4
  in5 : Inport  Port=5
  in6 : Inport  Port=6
  in7 : Inport  Port=7
  in8 : Inport  Port=8
  in9 : Inport  Port=9
  in10 : Inport  Port=10
  concatenate : xbsIndex_r4/Concat  num_inputs=10  dbl_ovrd=off  block_type=concat
  reinterpret{1..10} (10 alike) : xbsIndex_r4/Reinterpret  force_arith_type=on  arith_type=Unsigned  force_bin_pt=on  bin_pt=0  block_type=reinterpret
      reinterpret1 settings: infoedit="Changes signal type without altering the binary representation.   You can changed the signal between signed and unsigned, and relocate the binary point.<br><br>Hardware notes: In hardware this block costs nothing.<br><br>Example:  Suppose the input is 6 bits wide, signed, with 2 fractional bits, and the output is forced to unsigned with 0 fractional bits.  Then an input of -2.0 (1110.00 in binary 2's complement) becomes an output of 56 (111000 in binary)."
      reinterpret2 settings: infoedit="Changes signal type without altering the binary representation.   You can changed the signal between signed and unsigned, and relocate the binary point.<br><br>Hardware notes: In hardware this block costs nothing.<br><br>Example:  Suppose the input is 6 bits wide, signed, with 2 fractional bits, and the output is forced to unsigned with 0 fractional bits.  Then an input of -2.0 (1110.00 in binary 2's complement) becomes an output of 56 (111000 in binary)."
  bus_out : Outport
  wires:
  concatenate/1 -> bus_out/1
  in1/1 -> reinterpret1/1
  reinterpret1/1 -> concatenate/1
  in2/1 -> reinterpret2/1
  reinterpret2/1 -> concatenate/2
  in3/1 -> reinterpret3/1
  reinterpret3/1 -> concatenate/3
  in4/1 -> reinterpret4/1
  reinterpret4/1 -> concatenate/4
  in5/1 -> reinterpret5/1
  reinterpret5/1 -> concatenate/5
  in6/1 -> reinterpret6/1
  reinterpret6/1 -> concatenate/6
  in7/1 -> reinterpret7/1
  reinterpret7/1 -> concatenate/7
  in8/1 -> reinterpret8/1
  reinterpret8/1 -> concatenate/8
  in9/1 -> reinterpret9/1
  reinterpret9/1 -> concatenate/9
  in10/1 -> reinterpret10/1
  reinterpret10/1 -> concatenate/10
